simulink model "fb_linearises_control101"  (R2024a)
settings: Solver=VariableStepAuto  StartTime=0.0  StopTime=endtime  RelTol=1e-3
settings Model: Creator=barsr  LastModifiedBy=Anthony Rossiter
settings DebuggingCC: AlgebraicLoopMsg=none
settings RTWCC: GPUComputeCapability=3.5

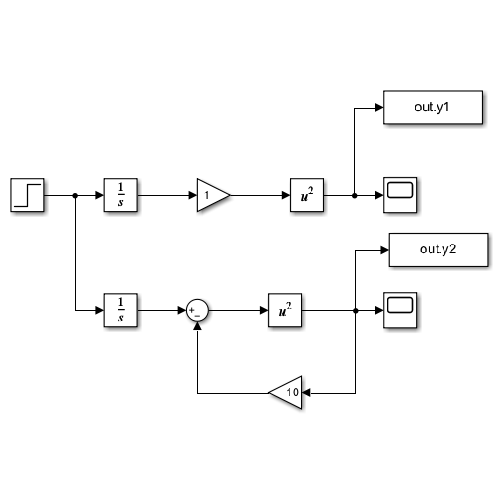
[thumbnail: Simulink's stored preview of the top-level diagram]
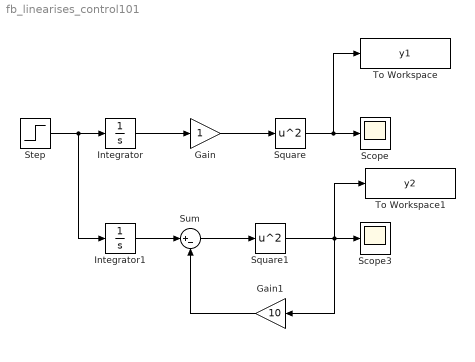
== system fb_linearises_control101 ==
  Gain : Gain
  Gain1 : Gain  Gain=10
  Integrator : Integrator
  Integrator1 : Integrator
  Scope : Scope
  Scope3 : Scope
  Square : Math  Operator=square
  Square1 : Math  Operator=square
  Step : Step  Time=0  SampleTime=0
  Sum : Sum  Inputs=|+-
  To Workspace : ToWorkspace  VariableName=y1  SaveFormat=Structure With Time  SampleTime=-1
  To Workspace1 : ToWorkspace  VariableName=y2  SaveFormat=Structure With Time  SampleTime=-1
  wires:
  Step/1 -> Integrator1/1, Integrator/1
  Integrator/1 -> Gain/1
  Gain/1 -> Square/1
  Square/1 -> To Workspace/1, Scope/1
  Integrator1/1 -> Sum/1
  Square1/1 -> To Workspace1/1, Gain1/1, Scope3/1
  Sum/1 -> Square1/1
  Gain1/1 -> Sum/2
